simulink model "D6"  (R2019b)
settings: Solver=FixedStepAuto  StartTime=0.0  StopTime=3  FixedStep=0.010000  RelTol=1e-3
libraries: dspsigops x2
settings Model: Creator=nahkusaidy  LastModifiedBy=nahkusaidy

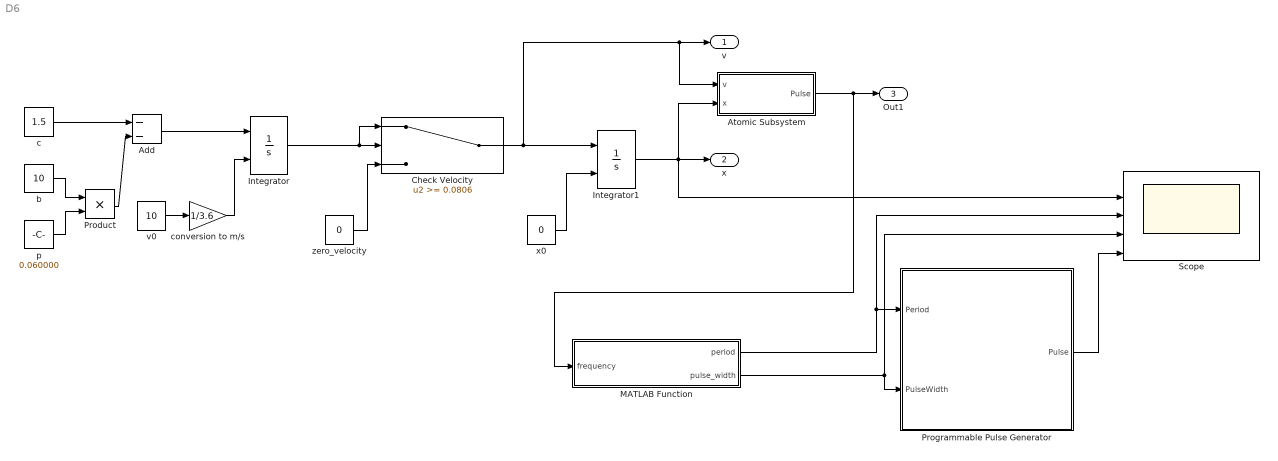
== system D6 ==
  Add : Sum  Inputs=--
  Atomic Subsystem : Subsystem  TreatAsAtomicUnit=on
  Check Velocity : Switch  Threshold=0.0806
  Integrator : Integrator  InitialConditionSource=external
  Integrator1 : Integrator  InitialConditionSource=external
  MATLAB Function : MATLAB Function  TreatAsAtomicUnit=on
  Product : Product
  Programmable Pulse Generator : Subsystem
  Scope : Scope  NumInputPorts=5
  b : Constant  Value=10
  c : Constant  Value=1.5
  conversion to m/s : Gain  Gain=1/3.6
  p : Constant  Value=0.060000
  v0 : Constant  Value=10
  x0 : Constant  Value=0
  "zero_velocity " : Constant  Value=0
  v : Outport
  "x " : Outport  Port=2
  Out1 : Outport  Port=3
  wires:
  Add/1 -> Integrator/1
  v0/1 -> conversion to m/s/1
  x0/1 -> Integrator1/2
  p/1 -> Product/2
  conversion to m/s/1 -> Integrator/2
  "zero_velocity "/1 -> Check Velocity/3
  Product/1 -> Add/2
  Integrator/1 -> Check Velocity/1, Check Velocity/2
  c/1 -> Add/1
  b/1 -> Product/1
  Integrator1/1 -> Scope/2, Atomic Subsystem/2(x), "x "/1
  Check Velocity/1 -> Atomic Subsystem/1("v "), v/1, Integrator1/1
  Atomic Subsystem/1(Pulse) -> MATLAB Function/1(frequency), Out1/1
  MATLAB Function/1(period) -> Scope/3, Programmable Pulse Generator/1(Period)
  Programmable Pulse Generator/1(Pulse) -> Scope/5
  MATLAB Function/2(pulse_width) -> Programmable Pulse Generator/2(PulseWidth), Scope/4

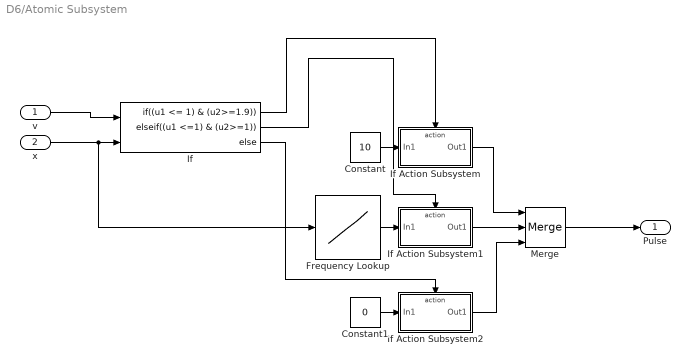
== system D6/Atomic Subsystem ==
  "v " : Inport
  x : Inport  Port=2
  Constant : Constant  Value=10
  Constant1 : Constant  Value=0
  Frequency Lookup : Lookup_n-D  NumberOfTableDimensions=1  BreakpointsForDimension1=[1,1.9]  Table=[1,9]  InternalRulePriority=Speed  RndMeth=Simplest  InputSameDT=on
  If : If  NumInputs=2  IfExpression=(u1 <= 1) & (u2>=1.9)  ElseIfExpressions=(u1 <=1) & (u2>=1)
  If Action Subsystem : Subsystem  TreatAsAtomicUnit=on
  If Action Subsystem1 : Subsystem  TreatAsAtomicUnit=on
  If Action Subsystem2 : Subsystem  TreatAsAtomicUnit=on
  Merge : Merge  Inputs=3
  Pulse : Outport
  wires:
  x/1 -> Frequency Lookup/1, If/2
  Constant1/1 -> If Action Subsystem2/1(In1)
  If/1 -> If Action Subsystem/Action
  Constant/1 -> If Action Subsystem/1(In1)
  If Action Subsystem2/1(Out1) -> Merge/3
  Frequency Lookup/1 -> If Action Subsystem1/1(In1)
  If Action Subsystem1/1(Out1) -> Merge/2
  If/3 -> If Action Subsystem2/Action
  If/2 -> If Action Subsystem1/Action
  If Action Subsystem/1(Out1) -> Merge/1
  "v "/1 -> If/1
  Merge/1 -> Pulse/1

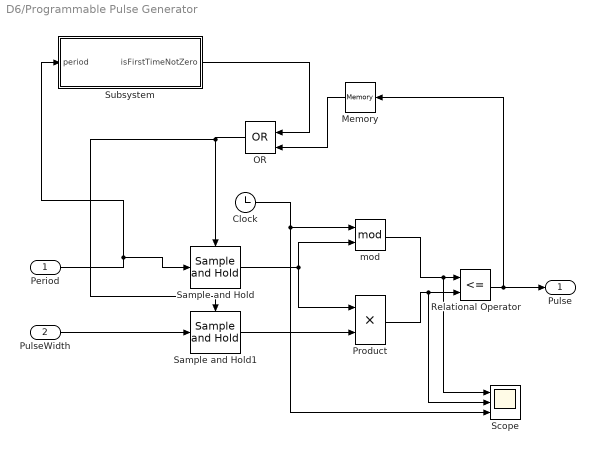
== system D6/Programmable Pulse Generator ==
  Period : Inport
  PulseWidth : Inport  Port=2
  Clock : Clock
  Memory : Memory
  OR : Logic  Operator=OR  IconShape=distinctive  AllPortsSameDT=off  OutDataTypeStr=boolean
  Product : Product  RndMeth=Zero
  Relational Operator : RelationalOperator  Operator=<=  RndMeth=Nearest
  Sample and Hold : dspsigops/Sample and Hold  trig=Rising edge  initCond=0  latchinput=off
  Sample and Hold1 : dspsigops/Sample and Hold  trig=Rising edge  initCond=0  latchinput=off
  Scope : Scope  NumInputPorts=3
  Subsystem : Subsystem
  mod : Math  Operator=mod  SaturateOnIntegerOverflow=on
  Pulse : Outport
  wires:
  Product/1 -> Scope/2, Relational Operator/2
  Relational Operator/1 -> Memory/1, Pulse/1
  mod/1 -> Scope/1, Relational Operator/1
  Period/1 -> Sample and Hold/1, Subsystem/1(period)
  Clock/1 -> Scope/3, mod/1
  Sample and Hold/1 -> Product/1, mod/2
  Sample and Hold1/1 -> Product/2
  PulseWidth/1 -> Sample and Hold1/1
  Memory/1 -> OR/2
  OR/1 -> Sample and Hold1/Trigger, Sample and Hold/Trigger
  Subsystem/1("isFirstTimeNotZero ") -> OR/1

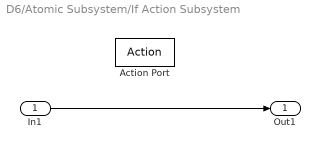
== system D6/Atomic Subsystem/If Action Subsystem ==
  In1 : Inport
  Action Port : ActionPort  ActionPortLabel=if((u1 <= 1) & (u2>=1.9))
  Out1 : Outport
  wires:
  In1/1 -> Out1/1

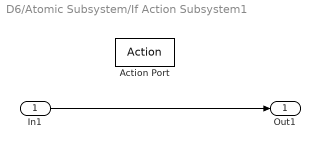
== system D6/Atomic Subsystem/If Action Subsystem1 ==
  In1 : Inport
  Action Port : ActionPort  ActionPortLabel=elseif( (u1 <=1) & (u2>=1))
  Out1 : Outport
  wires:
  In1/1 -> Out1/1

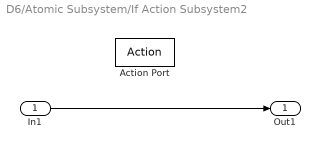
== system D6/Atomic Subsystem/If Action Subsystem2 ==
  In1 : Inport
  Action Port : ActionPort  ActionPortLabel=else
  Out1 : Outport
  wires:
  In1/1 -> Out1/1

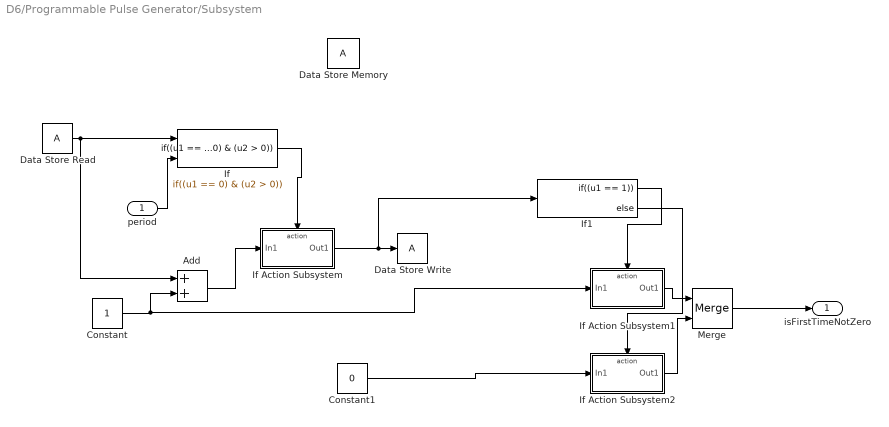
== system D6/Programmable Pulse Generator/Subsystem ==
  period : Inport
  Add : Sum
  Constant : Constant
  Constant1 : Constant  Value=0
  Data Store Memory : DataStoreMemory  ReadBeforeWriteMsg=warning  WriteAfterWriteMsg=warning  WriteAfterReadMsg=warning  ShowAdditionalParam=off
  Data Store Read : DataStoreRead
  Data Store Write : DataStoreWrite
  If : If  NumInputs=2  IfExpression=(u1 == 0) & (u2 > 0)  ShowElse=off
  If Action Subsystem : Subsystem  TreatAsAtomicUnit=on
  If Action Subsystem1 : Subsystem  TreatAsAtomicUnit=on
  If Action Subsystem2 : Subsystem  TreatAsAtomicUnit=on
  If1 : If  IfExpression=(u1 == 1)
  Merge : Merge
  "isFirstTimeNotZero " : Outport
  wires:
  Data Store Read/1 -> Add/1, If/1
  period/1 -> If/2
  If Action Subsystem/1(Out1) -> If1/1, Data Store Write/1
  If/1 -> If Action Subsystem/Action
  Add/1 -> If Action Subsystem/1(In1)
  Constant/1 -> If Action Subsystem1/1(In1), Add/2
  If1/1 -> If Action Subsystem1/Action
  If Action Subsystem1/1(Out1) -> Merge/1
  Merge/1 -> "isFirstTimeNotZero "/1
  If1/2 -> If Action Subsystem2/Action
  Constant1/1 -> If Action Subsystem2/1(In1)
  If Action Subsystem2/1(Out1) -> Merge/2

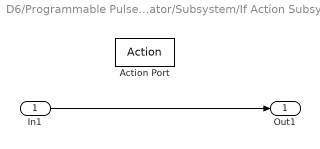
== system D6/Programmable Pulse Generator/Subsystem/If Action Subsystem ==
  In1 : Inport
  Action Port : ActionPort  ActionPortLabel=if((u1 == 0) & (u2 > 0))
  Out1 : Outport
  wires:
  In1/1 -> Out1/1

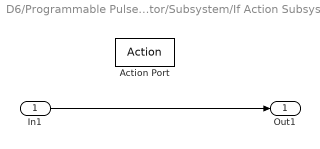
== system D6/Programmable Pulse Generator/Subsystem/If Action Subsystem1 ==
  In1 : Inport
  Action Port : ActionPort  ActionPortLabel=if((u1 == 1))
  Out1 : Outport
  wires:
  In1/1 -> Out1/1

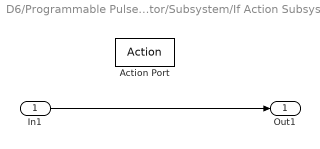
== system D6/Programmable Pulse Generator/Subsystem/If Action Subsystem2 ==
  In1 : Inport
  Action Port : ActionPort  ActionPortLabel=else
  Out1 : Outport
  wires:
  In1/1 -> Out1/1

== matlab function D6/MATLAB Function ==
  data: frequency input; period output; pulse_width output
function [period, pulse_width] = fcn(frequency)
%TEST_SQUARE Summary of this function goes here
%   Detailed explanation goes here
standard_pulse_width = 0.1; %second
period = 0;
if((frequency>=1) && (frequency <=9))
    period = 1/frequency;
    pulse_width = (standard_pulse_width/period); %pulse width 0.1
    
else
    period = 0;
    pulse_width = 0;
end
end
